simulink model "VisionModel_v5"  (Simulink 7.6)
settings: Solver=FixedStepDiscrete  StartTime=0.0  StopTime=0  RelTol=1e-3
values from neighbouring files (symbols this model uses):
  Iter_Segment_Thresh = 60    [VisionConstants.m]
  Scale_Down_B = 1    [VisionConstants.m]
  Scale_Down_G = 1    [VisionConstants.m]
  Scale_Down_H = 1    [VisionConstants.m]
  Scale_Down_R = 1    [VisionConstants.m]
  Scale_Down_S = 1    [VisionConstants.m]
  Scale_Down_V = 5    [VisionConstants.m]
  Scale_Forward_B = 0    [VisionConstants.m]
  Scale_Forward_G = 1    [VisionConstants.m]
  Scale_Forward_H = 1    [VisionConstants.m]
  Scale_Forward_R = 0    [VisionConstants.m]
  Scale_Forward_S = 1    [VisionConstants.m]
  Scale_Forward_V = 5    [VisionConstants.m]
undefined symbols (not defined in the file or in its folder): Rec, SDTV
libraries: vipconversions x4
settings Model: Creator=Administrator  LastModifiedBy=auvt
settings OptimizationCC: OptimizeModelRefInitCode=on
settings RTWCC: SystemTargetFile=ert.tlc  GenCodeOnly=on  TemplateMakefile=ert_default_tmf  PostCodeGenCommand=packNGo(buildInfo, {'packType' 'flat'})  Description=Real-Time Workshop Embedded Coder  GenerateReport=on  ProcessScript=ert_make_rtw_hook  IncludeHyperlinkInReport=on  LaunchReport=on  TargetLang=C++
settings CodeAppCC: IgnoreCustomStorageClasses=off
settings ERTTargetCC: MultiwordLength=2048  GenerateSampleERTMain=on  IncludeMdlTerminateFcn=off  ERTCustomFileTemplate=example_file_process.tlc  ConvertIfToSwitch=off

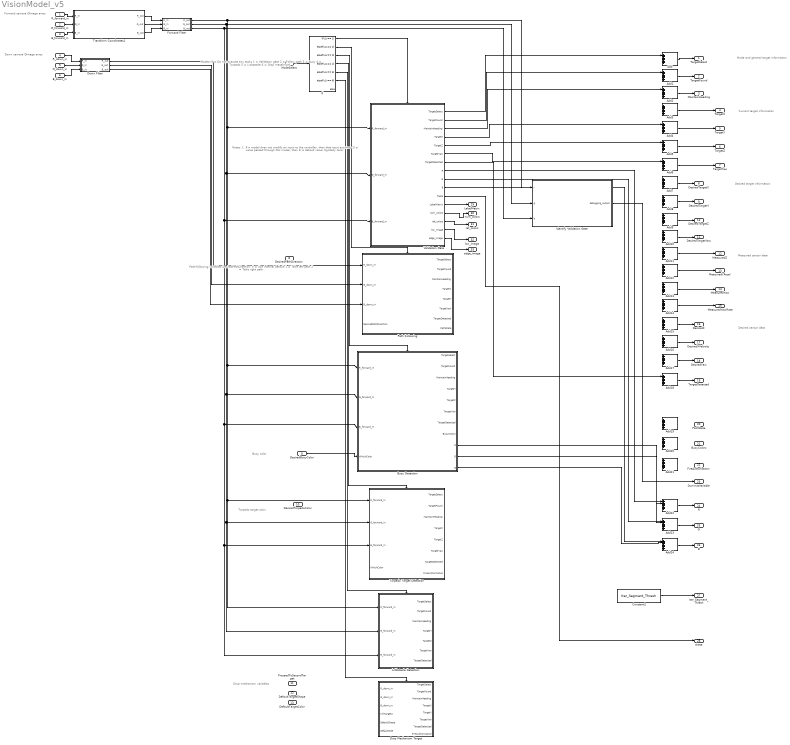
== system VisionModel_v5 ==
  note: Current target information
  note: Desired target information
  note: Measured sensor data
  note: Mode and general target information
  note: Desired sensor data
  note: Forward camera QImage array
  note: Modes:
      | 0 = Do not execute any tasks
      | 1 = Validation gate
      | 2 = Follow path
      | 3 = Buoy
      | 4 = Torpedo
      | 5 = L-obstacle
      | 6 = Drop mecahnism
  note: Path-following variables
      | DesiredPathDirection:
      | 0 = Use internal default
      | 1 = Take left path
      | 2 = Take right path
  note: Buoy color
  note: Torpedo target color
  note: Drop mechanism variables
  note: Down camera QImage array
  note: Notes:
      | 1. If a model does not modify an input to the controller,
      | then that input assumes 1) a value passed through this
      | model, then 2) a default value (typically zero)
  R_forward_in : Inport  PortDimensions=Forward_Camera_Dimensions
  G_forward_in : Inport  Port=2  PortDimensions=Forward_Camera_Dimensions
  B_forward_in : Inport  Port=3  PortDimensions=Forward_Camera_Dimensions
  R_down_in : Inport  Port=4  PortDimensions=Down_Camera_Dimensions
  G_down_in : Inport  Port=5  PortDimensions=Down_Camera_Dimensions
  B_down_in : Inport  Port=6  PortDimensions=Down_Camera_Dimensions
  ModeSelect : Inport  Port=7
  DesiredPathDirection : Inport  Port=8
  DesiredBuoyColor : Inport  Port=9
  DesiredTorpedoColor : Inport  Port=10
  ProceedToSecondTarget : Inport  Port=11
  DefaultTargetShape : Inport  Port=12
  DefaultTargetColor : Inport  Port=13
  Add{,1..24} (25 alike) : Sum  Inputs=++++++
  Buoy Detection : Subsystem  TreatAsAtomicUnit=on
  Constant2 : Constant  Value=Iter_Segment_Thresh  SampleTime=-1
  Down Filter : Subsystem
  Drop Mechanism Target : Subsystem  TreatAsAtomicUnit=on
  Forward Filter : Subsystem
  Identify Validation Gate : Stateflow chart  TreatAsAtomicUnit=on  SystemSampleTime=[1/30 0]
  If : If  IfExpression=u1 == 1  ElseIfExpressions=u1 == 2, u1 == 3, u1 == 4, u1 == 5, u1 == 6
  L-Obstacle Detection : Subsystem  TreatAsAtomicUnit=on
  Path Following : Subsystem  TreatAsAtomicUnit=on
  Torpedo Target Detection : Subsystem  TreatAsAtomicUnit=on
  Transform Coordinates1 : Stateflow chart  TreatAsAtomicUnit=on  SystemSampleTime=[1/30 0]
  Validation Gate : Subsystem  TreatAsAtomicUnit=on
  TargetSelect : Outport  OutDataTypeStr=double
  TargetFound : Outport  Port=2  OutDataTypeStr=double
  MaintainHeading : Outport  Port=3  OutDataTypeStr=double
  TargetX : Outport  Port=4  OutDataTypeStr=double
  TargetY : Outport  Port=5  OutDataTypeStr=double
  TargetZ : Outport  Port=6  OutDataTypeStr=double
  TargetYaw : Outport  Port=7  OutDataTypeStr=double
  DesiredTargetX : Outport  Port=8  OutDataTypeStr=double
  DesiredTargetY : Outport  Port=9  OutDataTypeStr=double
  DesiredTargetZ : Outport  Port=10  OutDataTypeStr=double
  DesiredTargetYaw : Outport  Port=11  OutDataTypeStr=double
  MeasuredZ : Outport  Port=12  OutDataTypeStr=double
  MeasuredYAccel : Outport  Port=13  OutDataTypeStr=double
  MeasuredYaw : Outport  Port=14  OutDataTypeStr=double
  MeasuredYawRate : Outport  Port=15  OutDataTypeStr=double
  DesiredZ : Outport  Port=16  OutDataTypeStr=double
  DesiredXVelocity : Outport  Port=17  OutDataTypeStr=double
  DesiredYaw : Outport  Port=18  OutDataTypeStr=double
  TargetDetected : Outport  Port=19  OutDataTypeStr=double
  PathState : Outport  Port=20  OutDataTypeStr=double
  BuoyColors : Outport  Port=21  OutDataTypeStr=double
  FireAuthorization : Outport  Port=22  OutDataTypeStr=double
  DummieVariable : Outport  Port=23  OutDataTypeStr=double
  R : Outport  Port=24  OutDataTypeStr=double
  G : Outport  Port=25  OutDataTypeStr=double
  B : Outport  Port=26  OutDataTypeStr=double
  Iter_Segment_Thresh : Outport  Port=27  OutDataTypeStr=double
  theta : Outport  Port=28  OutDataTypeStr=double
  LabelMatrix : Outport  Port=29
  num_colors : Outport  Port=30
  ref_colors : Outport  Port=31
  bw_image : Outport  Port=32
  edge_image : Outport  Port=33
  wires:
  ModeSelect/1 -> If/1
  If/2 -> Path Following/Action
  If/3 -> Buoy Detection/Action
  If/1 -> Validation Gate/Action
  If/4 -> Torpedo Target Detection/Action
  If/5 -> L-Obstacle Detection/Action
  If/6 -> Drop Mechanism Target/Action
  DesiredBuoyColor/1 -> Buoy Detection/4(WhichColor)
  Down Filter/1(R_out) -> Path Following/1(R_down_in)
  Down Filter/2(G_out) -> Path Following/2(G_down_in)
  Down Filter/3(B_out) -> Path Following/3(B_down_in)
  Add/1 -> TargetSelect/1
  Add1/1 -> TargetFound/1
  Add2/1 -> MaintainHeading/1
  Add3/1 -> TargetX/1
  Add4/1 -> TargetY/1
  Add5/1 -> TargetZ/1
  Add6/1 -> TargetYaw/1
  Add7/1 -> DesiredTargetX/1
  Add8/1 -> DesiredTargetY/1
  Add9/1 -> DesiredTargetZ/1
  Add10/1 -> DesiredTargetYaw/1
  Add11/1 -> MeasuredZ/1
  Add12/1 -> MeasuredYAccel/1
  Add13/1 -> MeasuredYaw/1
  Add14/1 -> MeasuredYawRate/1
  Add15/1 -> DesiredZ/1
  Add16/1 -> DesiredXVelocity/1
  Add17/1 -> DesiredYaw/1
  Forward Filter/2(G_out) -> Validation Gate/2(G_forward_in), Buoy Detection/2(G_forward_in), Torpedo Target Detection/2(G_forward_in), L-Obstacle Detection/2(G_forward_in), Identify Validation Gate/2(g)
  Forward Filter/3(B_out) -> Validation Gate/3(B_forward_in), Buoy Detection/3(B_forward_in), Torpedo Target Detection/3(B_forward_in), L-Obstacle Detection/3(B_forward_in), Identify Validation Gate/3(b)
  Forward Filter/1(R_out) -> Validation Gate/1(R_forward_in), Buoy Detection/1(R_forward_in), Torpedo Target Detection/1(R_forward_in), L-Obstacle Detection/1(R_forward_in), Identify Validation Gate/1(r)
  G_down_in/1 -> Down Filter/2(G_in)
  R_down_in/1 -> Down Filter/1(R_in)
  B_down_in/1 -> Down Filter/3(B_in)
  Validation Gate/5(TargetZ) -> Add5/1
  Validation Gate/4(TargetY) -> Add4/1
  Validation Gate/1(TargetSelect) -> Add/1
  Validation Gate/2(TargetFound) -> Add1/1
  Validation Gate/3(MaintainHeading) -> Add2/1
  Validation Gate/6(TargetYaw) -> Add6/1
  Validation Gate/7(TargetDetected) -> Add18/1
  Add18/1 -> TargetDetected/1
  Add22/1 -> R/1
  Add23/1 -> G/1
  Add24/1 -> B/1
  Validation Gate/8(R) -> Add22/1
  Validation Gate/9(G) -> Add23/1
  Validation Gate/10(B) -> Add24/1
  Identify Validation Gate/1(debugging_output) -> DummieVariable/1
  Buoy Detection/9(R) -> Add22/2
  Buoy Detection/11(B) -> Add24/2
  Buoy Detection/10(G) -> Add23/2
  Constant2/1 -> Iter_Segment_Thresh/1
  Validation Gate/11(theta) -> theta/1
  G_forward_in/1 -> Transform Coordinates1/2(G_in)
  R_forward_in/1 -> Transform Coordinates1/1(R_in)
  B_forward_in/1 -> Transform Coordinates1/3(B_in)
  Transform Coordinates1/1(R_out) -> Forward Filter/1(R_in)
  Transform Coordinates1/2(G_out) -> Forward Filter/2(G_in)
  Transform Coordinates1/3(B_out) -> Forward Filter/3(B_in)
  Validation Gate/12(LabelMatrix) -> LabelMatrix/1
  Validation Gate/13(num_colors) -> num_colors/1
  Validation Gate/14(ref_colors) -> ref_colors/1
  Validation Gate/15(bw_image) -> bw_image/1
  Validation Gate/16(edge_image) -> edge_image/1

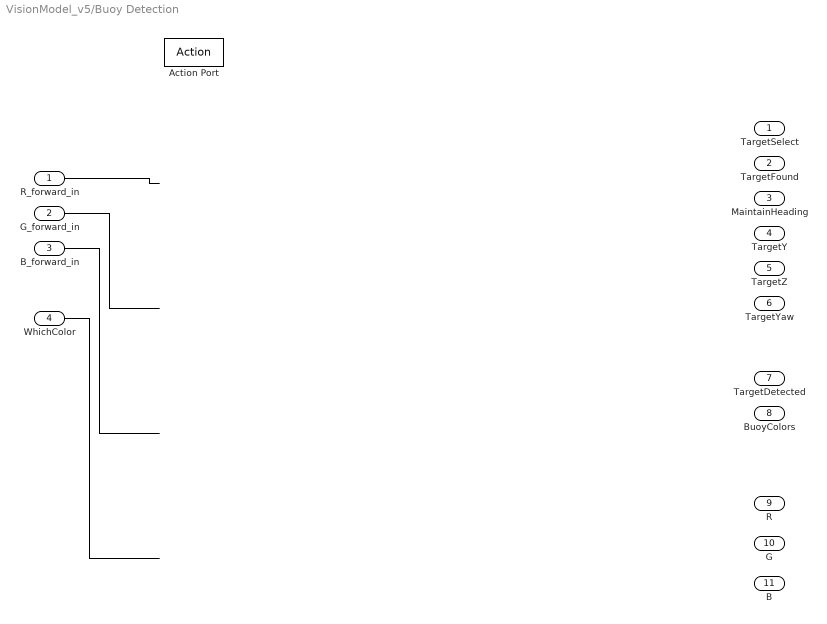
== system VisionModel_v5/Buoy Detection ==
  R_forward_in : Inport
  G_forward_in : Inport  Port=2
  B_forward_in : Inport  Port=3
  WhichColor : Inport  Port=4
  Action Port : ActionPort  ActionType=elseif
  TargetSelect : Outport  OutDataTypeStr=double
  TargetFound : Outport  Port=2  OutDataTypeStr=double
  MaintainHeading : Outport  Port=3  OutDataTypeStr=double
  TargetY : Outport  Port=4  OutDataTypeStr=double
  TargetZ : Outport  Port=5  OutDataTypeStr=double
  TargetYaw : Outport  Port=6  OutDataTypeStr=double
  TargetDetected : Outport  Port=7  OutDataTypeStr=double
  BuoyColors : Outport  Port=8  OutDataTypeStr=double
  R : Outport  Port=9  OutDataTypeStr=double
  G : Outport  Port=10  OutDataTypeStr=double
  B : Outport  Port=11  OutDataTypeStr=double
  wires:
  R_forward_in/1 -> ?
  G_forward_in/1 -> ?
  B_forward_in/1 -> ?
  WhichColor/1 -> ?
  ? -> TargetSelect/1
  ? -> TargetFound/1
  ? -> MaintainHeading/1
  ? -> TargetY/1
  ? -> TargetZ/1
  ? -> TargetYaw/1
  ? -> TargetDetected/1
  ? -> BuoyColors/1
  ? -> R/1
  ? -> G/1
  ? -> B/1

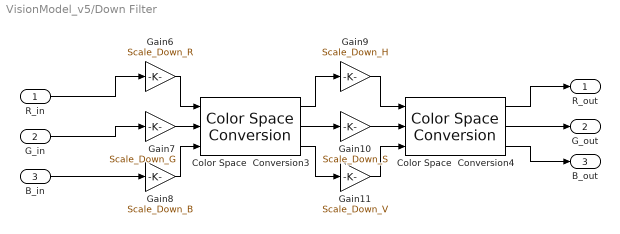
== system VisionModel_v5/Down Filter ==
  R_in : Inport  PortDimensions=Down_Camera_Dimensions
  G_in : Inport  Port=2  PortDimensions=Down_Camera_Dimensions
  B_in : Inport  Port=3  PortDimensions=Down_Camera_Dimensions
  Color Space  Conversion3 : vipconversions/Color Space  Conversion  conversion=Obsolete  conversionActive=R'G'B' to HSV  wp_str=D50  rec=Rec. 601 (SDTV)  sys=1125/60/2:1  imagePorts=Separate color signals
  Color Space  Conversion4 : vipconversions/Color Space  Conversion  conversion=Obsolete  conversionActive=HSV to R'G'B'  wp_str=D50  rec=Rec. 601 (SDTV)  sys=1125/60/2:1  imagePorts=Separate color signals
  Gain10 : Gain  Gain=Scale_Down_S
  Gain11 : Gain  Gain=Scale_Down_V
  Gain6 : Gain  Gain=Scale_Down_R
  Gain7 : Gain  Gain=Scale_Down_G
  Gain8 : Gain  Gain=Scale_Down_B
  Gain9 : Gain  Gain=Scale_Down_H
  R_out : Outport  OutDataTypeStr=double
  G_out : Outport  Port=2  OutDataTypeStr=double
  B_out : Outport  Port=3  OutDataTypeStr=double
  wires:
  Gain6/1 -> Color Space  Conversion3/1
  Gain7/1 -> Color Space  Conversion3/2
  Gain8/1 -> Color Space  Conversion3/3
  Color Space  Conversion3/1 -> Gain9/1
  Color Space  Conversion3/2 -> Gain10/1
  Color Space  Conversion3/3 -> Gain11/1
  Gain9/1 -> Color Space  Conversion4/1
  Gain10/1 -> Color Space  Conversion4/2
  Gain11/1 -> Color Space  Conversion4/3
  R_in/1 -> Gain6/1
  G_in/1 -> Gain7/1
  B_in/1 -> Gain8/1
  Color Space  Conversion4/1 -> R_out/1
  Color Space  Conversion4/2 -> G_out/1
  Color Space  Conversion4/3 -> B_out/1

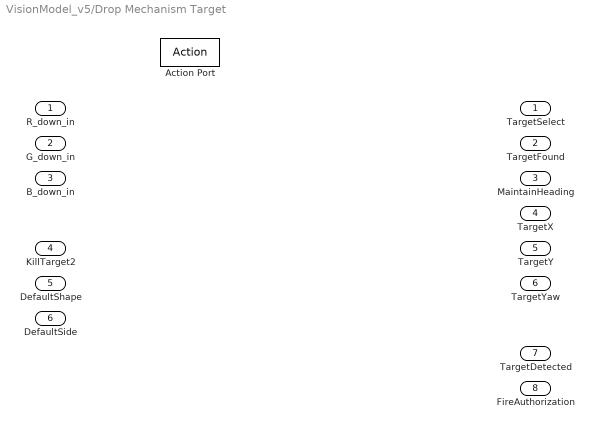
== system VisionModel_v5/Drop Mechanism Target ==
  R_down_in : Inport
  G_down_in : Inport  Port=2
  B_down_in : Inport  Port=3
  KillTarget2 : Inport  Port=4
  DefaultShape : Inport  Port=5
  DefaultSide : Inport  Port=6
  Action Port : ActionPort  ActionType=elseif
  TargetSelect : Outport  OutDataTypeStr=double
  TargetFound : Outport  Port=2  OutDataTypeStr=double
  MaintainHeading : Outport  Port=3  OutDataTypeStr=double
  TargetX : Outport  Port=4  OutDataTypeStr=double
  TargetY : Outport  Port=5  OutDataTypeStr=double
  TargetYaw : Outport  Port=6  OutDataTypeStr=double
  TargetDetected : Outport  Port=7  OutDataTypeStr=double
  FireAuthorization : Outport  Port=8  OutDataTypeStr=double

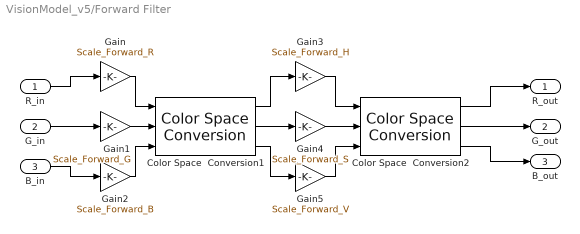
== system VisionModel_v5/Forward Filter ==
  R_in : Inport  PortDimensions=Forward_Camera_Dimensions
  G_in : Inport  Port=2  PortDimensions=Forward_Camera_Dimensions
  B_in : Inport  Port=3  PortDimensions=Forward_Camera_Dimensions
  Color Space  Conversion1 : vipconversions/Color Space  Conversion  conversion=Obsolete  conversionActive=R'G'B' to HSV  wp_str=D50  rec=Rec. 601 (SDTV)  sys=1125/60/2:1  imagePorts=Separate color signals
  Color Space  Conversion2 : vipconversions/Color Space  Conversion  conversion=Obsolete  conversionActive=HSV to R'G'B'  wp_str=D50  rec=Rec. 601 (SDTV)  sys=1125/60/2:1  imagePorts=Separate color signals
  Gain : Gain  Gain=Scale_Forward_R
  Gain1 : Gain  Gain=Scale_Forward_G
  Gain2 : Gain  Gain=Scale_Forward_B
  Gain3 : Gain  Gain=Scale_Forward_H
  Gain4 : Gain  Gain=Scale_Forward_S
  Gain5 : Gain  Gain=Scale_Forward_V
  R_out : Outport  OutDataTypeStr=double
  G_out : Outport  Port=2  OutDataTypeStr=double
  B_out : Outport  Port=3  OutDataTypeStr=double
  wires:
  R_in/1 -> Gain/1
  G_in/1 -> Gain1/1
  B_in/1 -> Gain2/1
  Gain/1 -> Color Space  Conversion1/1
  Gain1/1 -> Color Space  Conversion1/2
  Gain2/1 -> Color Space  Conversion1/3
  Color Space  Conversion1/1 -> Gain3/1
  Color Space  Conversion1/2 -> Gain4/1
  Color Space  Conversion1/3 -> Gain5/1
  Gain3/1 -> Color Space  Conversion2/1
  Gain4/1 -> Color Space  Conversion2/2
  Gain5/1 -> Color Space  Conversion2/3
  Color Space  Conversion2/1 -> R_out/1
  Color Space  Conversion2/2 -> G_out/1
  Color Space  Conversion2/3 -> B_out/1

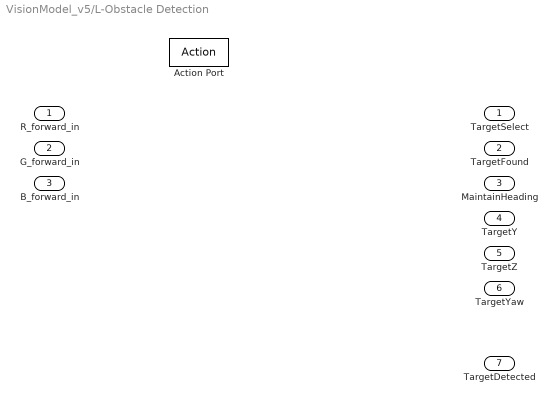
== system VisionModel_v5/L-Obstacle Detection ==
  R_forward_in : Inport
  G_forward_in : Inport  Port=2
  B_forward_in : Inport  Port=3
  Action Port : ActionPort  ActionType=elseif
  TargetSelect : Outport  OutDataTypeStr=double
  TargetFound : Outport  Port=2  OutDataTypeStr=double
  MaintainHeading : Outport  Port=3  OutDataTypeStr=double
  TargetY : Outport  Port=4  OutDataTypeStr=double
  TargetZ : Outport  Port=5  OutDataTypeStr=double
  TargetYaw : Outport  Port=6  OutDataTypeStr=double
  TargetDetected : Outport  Port=7  OutDataTypeStr=double

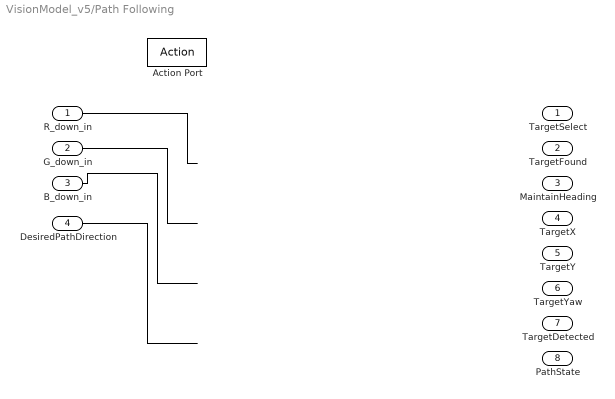
== system VisionModel_v5/Path Following ==
  R_down_in : Inport
  G_down_in : Inport  Port=2
  B_down_in : Inport  Port=3
  DesiredPathDirection : Inport  Port=4
  Action Port : ActionPort  ActionType=elseif
  TargetSelect : Outport  OutDataTypeStr=double
  TargetFound : Outport  Port=2  OutDataTypeStr=double
  MaintainHeading : Outport  Port=3  OutDataTypeStr=double
  TargetX : Outport  Port=4  OutDataTypeStr=double
  TargetY : Outport  Port=5  OutDataTypeStr=double
  TargetYaw : Outport  Port=6  OutDataTypeStr=double
  TargetDetected : Outport  Port=7  OutDataTypeStr=double
  PathState : Outport  Port=8  OutDataTypeStr=double
  wires:
  R_down_in/1 -> ?
  G_down_in/1 -> ?
  B_down_in/1 -> ?
  DesiredPathDirection/1 -> ?

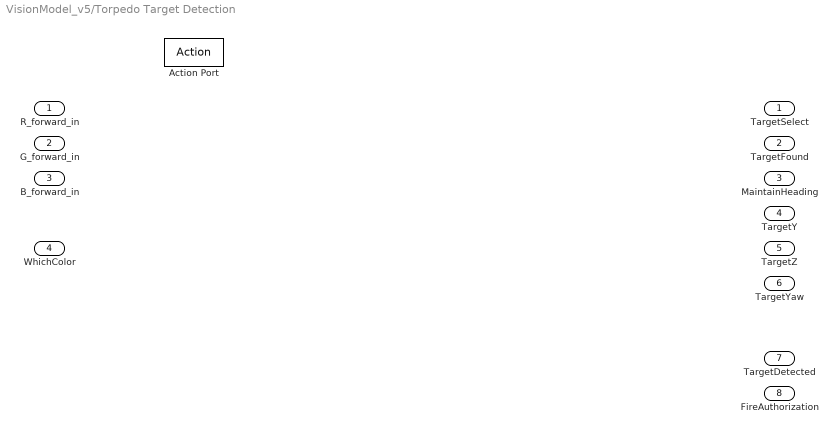
== system VisionModel_v5/Torpedo Target Detection ==
  R_forward_in : Inport
  G_forward_in : Inport  Port=2
  B_forward_in : Inport  Port=3
  WhichColor : Inport  Port=4
  Action Port : ActionPort  ActionType=elseif
  TargetSelect : Outport  OutDataTypeStr=double
  TargetFound : Outport  Port=2  OutDataTypeStr=double
  MaintainHeading : Outport  Port=3  OutDataTypeStr=double
  TargetY : Outport  Port=4  OutDataTypeStr=double
  TargetZ : Outport  Port=5  OutDataTypeStr=double
  TargetYaw : Outport  Port=6  OutDataTypeStr=double
  TargetDetected : Outport  Port=7  OutDataTypeStr=double
  FireAuthorization : Outport  Port=8  OutDataTypeStr=double

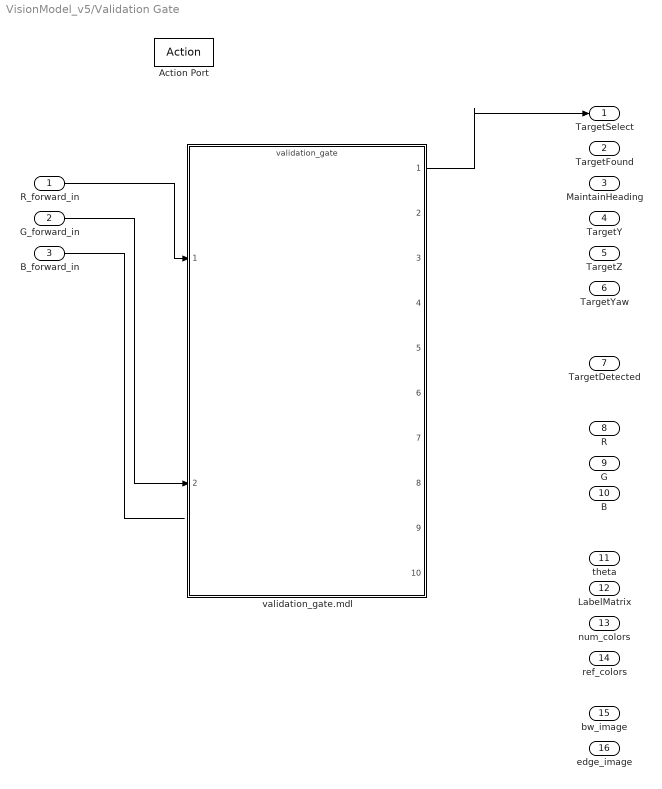
== system VisionModel_v5/Validation Gate ==
  R_forward_in : Inport
  G_forward_in : Inport  Port=2
  B_forward_in : Inport  Port=3
  Action Port : ActionPort  ActionType=then
  validation_gate.mdl : ModelReference  ModelNameDialog=validation_gate  SimulationMode=Accelerator  ModelReferenceVersion=1.1372  CopyOfModelName=validation_gate
  TargetSelect : Outport  OutDataTypeStr=double
  TargetFound : Outport  Port=2  OutDataTypeStr=double
  MaintainHeading : Outport  Port=3  OutDataTypeStr=double
  TargetY : Outport  Port=4  OutDataTypeStr=double
  TargetZ : Outport  Port=5  OutDataTypeStr=double
  TargetYaw : Outport  Port=6  OutDataTypeStr=double
  TargetDetected : Outport  Port=7  OutDataTypeStr=double
  R : Outport  Port=8  OutDataTypeStr=double
  G : Outport  Port=9  OutDataTypeStr=double
  B : Outport  Port=10  OutDataTypeStr=double
  theta : Outport  Port=11  OutDataTypeStr=double
  LabelMatrix : Outport  Port=12
  num_colors : Outport  Port=13
  ref_colors : Outport  Port=14
  bw_image : Outport  Port=15
  edge_image : Outport  Port=16
  wires:
  R_forward_in/1 -> validation_gate.mdl/1
  G_forward_in/1 -> validation_gate.mdl/2
  B_forward_in/1 -> ?
  ? -> TargetDetected/1
  ? -> TargetY/1
  ? -> TargetZ/1
  validation_gate.mdl/1 -> TargetSelect/1
  ? -> TargetFound/1
  ? -> MaintainHeading/1
  ? -> TargetYaw/1
  ? -> R/1
  ? -> G/1
  ? -> B/1
  ? -> theta/1
  ? -> LabelMatrix/1
  ? -> num_colors/1
  ? -> ref_colors/1
  ? -> bw_image/1
  ? -> edge_image/1

== matlab function Identify Validation Gate ==
  data: r input double; g input double; debugging_output output double; b input double
function debugging_output = dummie_function(r, g, b)
%#eml


debugging_output = sqrt(r(50,50)^2 + g(50,50)^2 + b(50,50)^2);

%debugging_output = max(max(max(g)));

return

== matlab function Transform Coordinates1 ==
  data: R_in input double; G_in input double; R_out output double; G_out output double; B_in input double; B_out output double
function [R_out, G_out, B_out] = rangeImage(R_in, G_in, B_in)
% Ensure the image components are between 0 and newMax

newMax = 1;

R_out = R_in;
G_out = G_in;
B_out = B_in;

normalizeValue = max(max(R_in));
if( normalizeValue <= 1 )
    normalizeValue = 1;
else
    normalizeValue = 255;
end

[rows, cols] = size(R_in);


for r = 1:rows
    for c = 1:cols
        
        if( R_in(r,c) == 0 )
            R_out(r,c) = 0;
        else
            R_out(r,c) = newMax*R_in(r,c)/normalizeValue;
        end
        if( G_in(r,c) == 0 )
            G_out(r,c) = 0;
        else
            G_out(r,c) = newMax*G_in(r,c)/normalizeValue;
        end
        if( B_in(r,c) == 0 )
            B_out(r,c) = 0;
        else
            B_out(r,c) = newMax*B_in(r,c)/normalizeValue;
        end
        
    end
end


return
